simulink subsystem "F550_Adam_CA"  (R2024a)
settings: Solver=VariableStepAuto  StartTime=0.0  StopTime=10.0  RelTol=1e-3
settings Model: Creator=UASG  LastModifiedBy=sslee

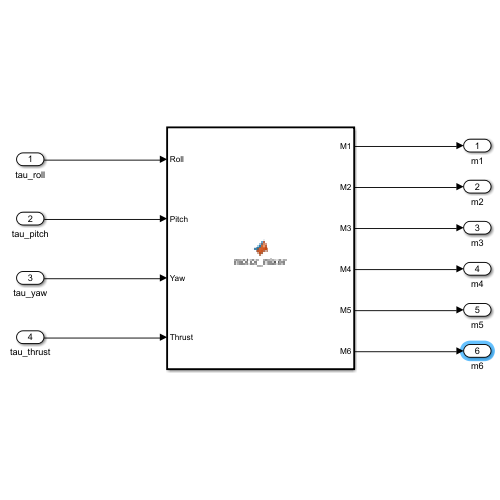
[thumbnail: Simulink's stored preview of the top-level diagram]
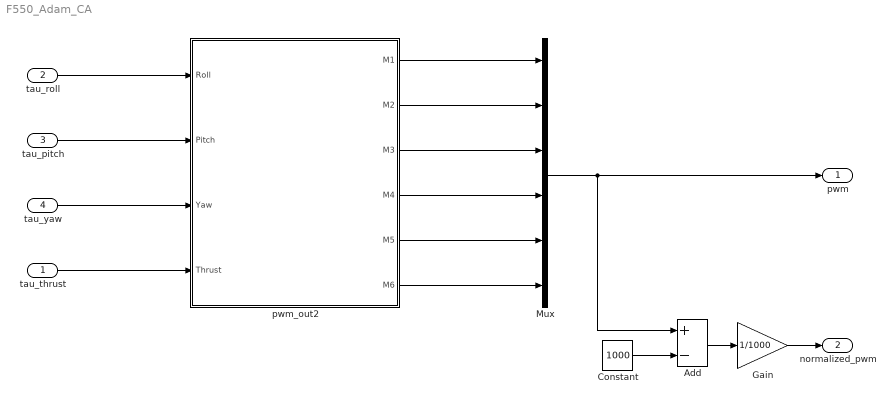
== system F550_Adam_CA ==
  tau_thrust : Inport
  tau_roll : Inport  Port=2
  tau_pitch : Inport  Port=3
  tau_yaw : Inport  Port=4
  Add : Sum  Inputs=+-
  Constant : Constant  Value=1000
  Gain : Gain  Gain=1/1000
  Mux : Mux  Inputs=6
  pwm_out2 : MATLAB Function  SystemSampleTime=0.004
  pwm : Outport
  normalized_pwm : Outport  Port=2
  wires:
  tau_roll/1 -> pwm_out2/1(Roll)
  tau_pitch/1 -> pwm_out2/2(Pitch)
  tau_yaw/1 -> pwm_out2/3(Yaw)
  tau_thrust/1 -> pwm_out2/4(Thrust)
  pwm_out2/1(M1) -> Mux/1
  pwm_out2/2(M2) -> Mux/2
  pwm_out2/3(M3) -> Mux/3
  pwm_out2/4(M4) -> Mux/4
  pwm_out2/5(M5) -> Mux/5
  pwm_out2/6(M6) -> Mux/6
  Mux/1 -> pwm/1, Add/1
  Constant/1 -> Add/2
  Add/1 -> Gain/1
  Gain/1 -> normalized_pwm/1

== matlab function F550_Adam_CA/pwm_out2 ==
  data: Roll input; M1 output; Pitch input; Yaw input; Thrust input; M2 output; M3 output; M4 output; M5 output; M6 output
function [M1, M2, M3, M4, M5, M6] = motor_mixer(Roll, Pitch, Yaw, Thrust)
%Function description:
%  Control allocation. The quadrotor type is X-configuration,
%  and the airframe is as follows:
%3↓   1↑
 %  \ /
 %  / \
 %2↑   4↓
%Input：
%  Roll, Pitch, Yaw: attitude controller output.
%  Thrust

idle_PWM = 1000;
scale = 1000;
scale_att = scale*Thrust;

% M1 = uint16(Thrust*scale + (- Roll + Pitch + Yaw) * scale_att + idle_PWM);
% M2 = uint16(Thrust*scale + (Roll - Pitch + Yaw) * scale_att + idle_PWM);
% M3 = uint16(Thrust*scale + (Roll + Pitch - Yaw) * scale_att + idle_PWM);
% M4 = uint16(Thrust*scale + (- Roll - Pitch - Yaw) * scale_att + idle_PWM);

% Hex X
% M1 = ((Pitch + Roll / 2 - Yaw) * Thrust / 2 + Thrust) * 1000 + idle_PWM;
% M2 = ((Pitch - Roll / 2 + Yaw) * Thrust / 2 + Thrust) * 1000 + idle_PWM;
% M3 = ((-Roll - Yaw) * Thrust / 2 + Thrust) * 1000 + idle_PWM;
% M4 = ((-Pitch - Roll / 2 + Yaw) * Thrust / 2 + Thrust) * 1000 + idle_PWM;
% M5 = ((-Pitch + Roll / 2 - Yaw) * Thrust / 2 + Thrust) * 1000 + idle_PWM;
% M6 = ((Roll + Yaw) * Thrust / 2 + Thrust) * 1000 + idle_PWM;
% M7 = 1000;
% M8 = 1000;

% Hex X (From Adam)
M1 = uint16(single(((-Roll - Yaw) * Thrust / 3 + Thrust) * single(1000))) + idle_PWM;
M2 = uint16(single(((Roll + Yaw) * Thrust / 3 + Thrust) * single(1000))) + idle_PWM;
M3 = uint16(single(((Pitch + (Roll / 2) - Yaw) * Thrust / 3 + Thrust) * single(1000))) + idle_PWM;
M4 = uint16(single(((-Pitch - (Roll / 2) + Yaw) * Thrust / 3 + Thrust) * single(1000))) + idle_PWM;
M5 = uint16(single(((Pitch - (Roll / 2) + Yaw) * Thrust / 3 + Thrust) * single(1000))) + idle_PWM;
M6 = uint16(single(((-Pitch + (Roll / 2) - Yaw) * Thrust / 3 + Thrust) * single(1000))) + idle_PWM;

% Hex X (Version 2)
% Roll/Yaw
% M1 = ((-Roll - Yaw) * Thrust / 2 + Thrust) * 1000 + idle_PWM;
% M2 = ((Roll + Yaw) * Thrust / 2 + Thrust) * 1000 + idle_PWM;
% % + Pitch/Roll
% M6 = ((Pitch + Roll / 2 - Yaw) * Thrust / 2 + Thrust) * 1000 + idle_PWM;
% M4 = ((Pitch - Roll / 2 + Yaw) * Thrust / 2 + Thrust) * 1000 + idle_PWM;
% % - Pitch/Roll
% M5 = ((-Pitch - Roll / 2 + Yaw) * Thrust / 2 + Thrust) * 1000 + idle_PWM;
% M3 = ((-Pitch + Roll / 2 - Yaw) * Thrust / 2 + Thrust) * 1000 + idle_PWM;
